simulink model "exam9_sim"  (R2023b)
settings: Solver=VariableStepAuto  StartTime=0.0  StopTime=10.0  RelTol=1e-3
settings Model: Creator=laptop  LastModifiedBy=maros-pc

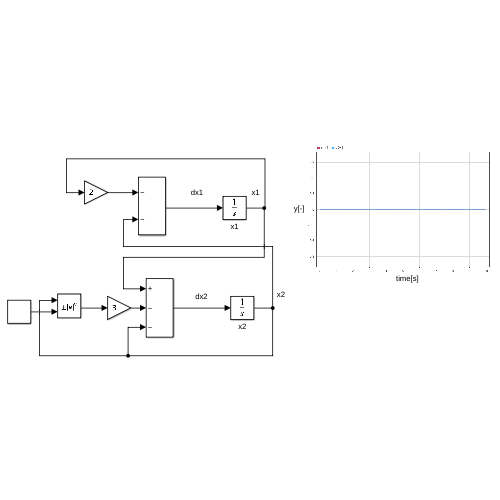
[thumbnail: Simulink's stored preview of the top-level diagram]
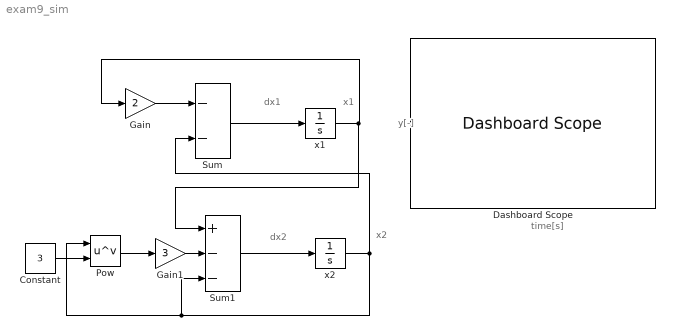
== system exam9_sim ==
  note: time[s]
  note: y[-]
  note: x1
  note: x2
  note: dx1
  note: dx2
  Constant : Constant  Value=3
  Dashboard Scope : DashboardScope
  Gain : Gain  Gain=2
  Gain1 : Gain  Gain=3
  Pow : Math  Operator=pow  SignedPower=on  RndMeth=Zero
  Sum : Sum  Inputs=--
  Sum1 : Sum  Inputs=+--
  x1 : Integrator
  x2 : Integrator
  wires:
  Gain/1 -> Sum/1
  Sum/1 -> x1/1
  x1/1 -> Sum1/1, Gain/1
  Sum1/1 -> x2/1
  Gain1/1 -> Sum1/2
  x2/1 -> Sum1/3, Pow/1, Sum/2
  Pow/1 -> Gain1/1
  Constant/1 -> Pow/2
